simulink model "rk"  (R2018b)
settings: Solver=ode4  StartTime=0.0  StopTime=1  FixedStep=0.01  RelTol=1e-3
settings Model: Creator=q5461  LastModifiedBy=q5461

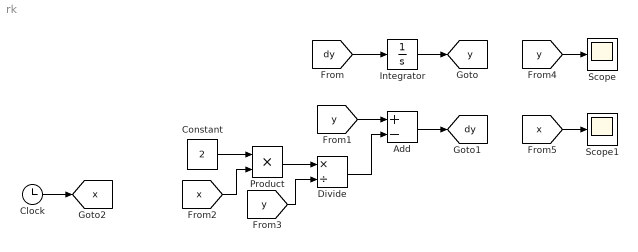
== system rk ==
  Add : Sum  Inputs=+-
  Clock : Clock
  Constant : Constant  Value=2
  Divide : Product  Inputs=*/
  Integrator : Integrator  InitialCondition=1
  Product : Product
  Scope : Scope
  Scope1 : Scope
  tag scope: dy=global, x=global, y=global
  wires:
  Integrator/1 -> [y]
  [dy] -> Integrator/1
  [y] -> Add/1
  Constant/1 -> Product/1
  [x] -> Product/2
  Product/1 -> Divide/1
  [y] -> Divide/2
  Divide/1 -> Add/2
  Add/1 -> [dy]
  [y] -> Scope/1
  [x] -> Scope1/1
  Clock/1 -> [x]
